simulink model "DynamicTF_OP"  (R2021b)
settings: Solver=FixedStepAuto  StartTime=0.0  StopTime=500  FixedStep=1  RelTol=1e-3
settings Model: Creator=ismt  LastModifiedBy=ismt
settings DataIOCC: SaveFormat=Array  ReturnWorkspaceOutputs=off

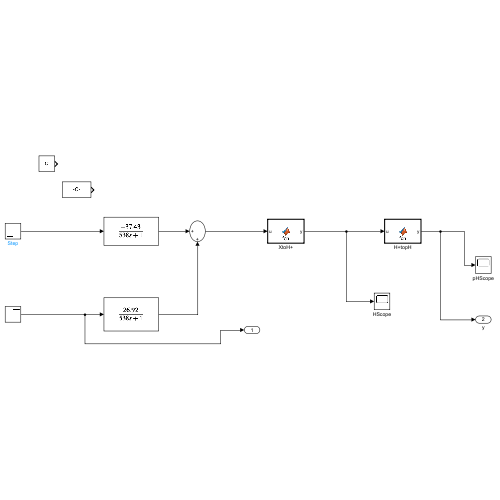
[thumbnail: Simulink's stored preview of the top-level diagram]
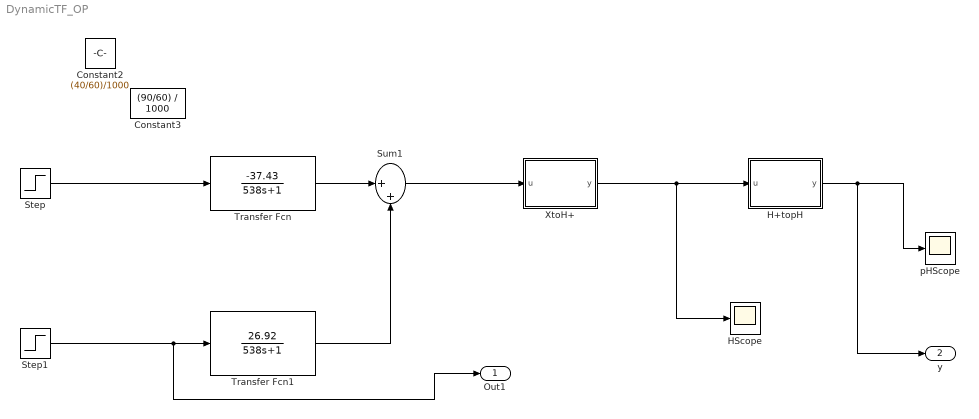
== system DynamicTF_OP ==
  Constant2 : Constant  Value=(40/60)/1000
  Constant3 : Constant  Value=(90/60) / 1000
  H+topH : MATLAB Function  TreatAsAtomicUnit=on
  HScope : Scope
  Step : Step  Time=205  After=0  SampleTime=0
  Step1 : Step  Time=205  After=(57/60) / 1000  SampleTime=0
  Sum1 : Sum  Inputs=|++
  Transfer Fcn : TransferFcn  Numerator=[-37.43]  Denominator=[538 1]
  Transfer Fcn1 : TransferFcn  Numerator=[26.92]  Denominator=[538 1]
  XtoH+ : MATLAB Function  TreatAsAtomicUnit=on
  pHScope : Scope
  Out1 : Outport
  y : Outport  Port=2
  wires:
  Step/1 -> Transfer Fcn/1
  Step1/1 -> Out1/1, Transfer Fcn1/1
  Transfer Fcn1/1 -> Sum1/2
  H+topH/1(y) -> y/1, pHScope/1
  Transfer Fcn/1 -> Sum1/1
  Sum1/1 -> XtoH+/1(u)
  XtoH+/1(y) -> HScope/1, H+topH/1(u)

== matlab function DynamicTF_OP/XtoH+ ==
  data: u input; y output
function y = fcn(u)

y = sqrt(((u^2)/4) + 10^(-14))-(u/2);
end

== matlab function DynamicTF_OP/H+topH ==
  data: u input; y output
function y = fcn(u)

y = -log10(u);
end
